simulink model "crane_DevDriv_2016a"  (R2016a)
settings: Solver=ode5  StartTime=0.0  StopTime=inf  FixedStep=0.01  RelTol=1e-3
values from neighbouring files (symbols this model uses):
  start_course = 1    [a_1_run_script.m]
  total_waypoints = length(waypoints_list)    [a_1_run_script.m]
undefined symbols (not defined in the file or in its folder): Crane3D_RangeBit, Crane3D_ScaleCoeff, xwaypoints, ywaypoints
undefined symbols (not defined in the file): RTDAC4PCIBaseAddress
libraries: simulink x2
settings Model: SimulationMode=external  ExtModeTrigDuration=5000  Creator=The MathWorks Inc.  LastModifiedBy=nadeen
settings DataIOCC: SaveFormat=StructureWithTime  SignalLoggingSaveFormat=ModelDataLogs  SignalLoggingName=logsOut
settings OptimizationCC: ExpressionDepthLimit=2147483647  InitFltsAndDblsToZero=on  EfficientMapNaN2IntZero=off
settings DebuggingCC: UnderspecifiedInitializationDetection=Classic  MergeDetectMultiDrivingBlocksExec=none  SignalResolutionControl=TryResolveAllWithWarning  FcnCallInpInsideContextMsg=EnableAllAsWarning  StateNameClashWarn=warning
settings HardwareCC: TargetBitPerLong=64  TargetBitPerPointer=64  TargetIntDivRoundTo=Zero  TargetEndianess=LittleEndian  TargetWordSize=64  TargetHWDeviceType=Intel->x86-64
settings ModelReferenceCC: PropagateSignalLabelsOutOfModel=off
settings RTWCC: SystemTargetFile=sldrt.tlc  TemplateMakefile=sldrt.tmf  Description=Simulink Desktop Real-Time  RTWCompilerOptimization=on
settings CodeAppCC: MaxIdLength=95
settings SimulinkDesktopRealTimeCC: TargetPreCompLibLocation=C:\Program Files\MATLAB\R2016b\toolbox\sldrt\lib\win64  TargetLangStandard=C89/C90 (ANSI)  SupportVariableSizeSignals=off
settings ConfigComp: CovSFcnEnable=off

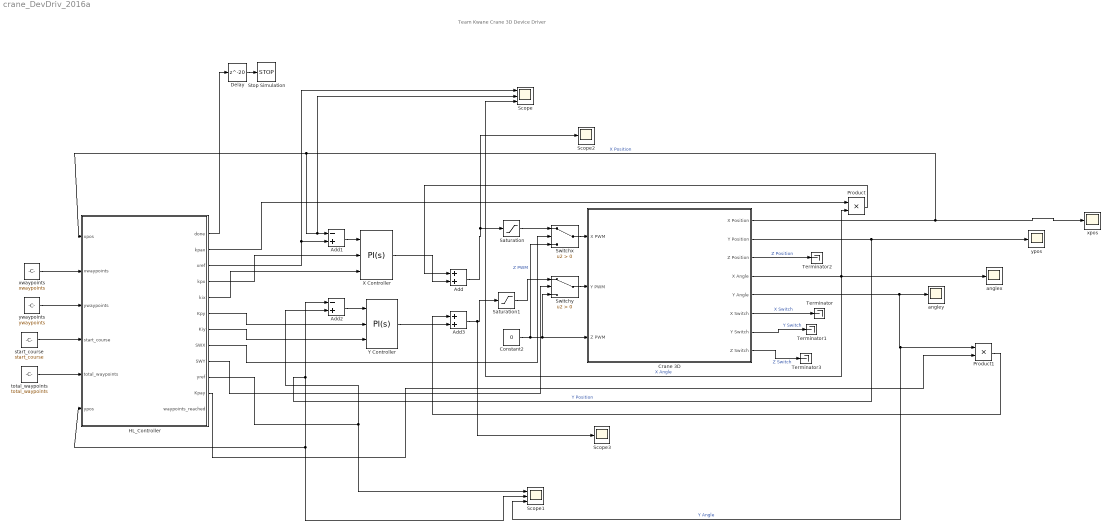
== system crane_DevDriv_2016a ==
  note: Team Kwane Crane 3D Device Driver
  Add : Sum
  Add1 : Sum  Inputs=-+
  Add2 : Sum  Inputs=-+
  Add3 : Sum
  Constant2 : Constant  Value=0
  Crane 3D : Subsystem  mask{BaseAddress=RTDAC4PCIBaseAddress, T0=0.01}
      mask prompts: BaseAddress "Base Address:"; T0 "Samping Period:"
      mask Display: image(imread('crane.jpeg'))
  Delay : Delay  DelayLength=20
  HL_Controller : Stateflow chart  TreatAsAtomicUnit=on
      settings: PermitHierarchicalResolution=ParametersOnly
  Product : Product
  Product1 : Product
  Saturation : Saturate  UpperLimit=0.8  LowerLimit=-0.8
  Saturation1 : Saturate  UpperLimit=0.8  LowerLimit=-0.8
  Scope : Scope  NumInputPorts=3
  Scope1 : Scope  NumInputPorts=3
  Scope2 : Scope
  Scope3 : Scope
  Stop Simulation : Stop
  Switchx : Switch  Criteria=u2 > Threshold
  Switchy : Switch  Criteria=u2 > Threshold
  Terminator{,1..3} (4 alike) : Terminator
  X Controller : simulink/Continuous/PID Controller  Controller=PI  TimeDomain=Continuous-time  SampleTime=-1  IntegratorMethod=Forward Euler  FilterMethod=Forward Euler  Form=Parallel  UseFilter=on  ControllerParametersSource=external  P=1  I=1  D=0  N=100  InitialConditionSource=internal  InitialConditionForIntegrator=0  InitialConditionForFilter=0  ExternalReset=none  LimitOutput=off  UpperSaturationLimit=inf  LowerSaturationLimit=-inf  LinearizeAsGain=on  AntiWindupMode=none  Kb=1  TrackingMode=off  Kt=1  PParamMin=[]  PParamMax=[]  IParamMin=[]  IParamMax=[]  DParamMin=[]  DParamMax=[]  NParamMin=[]  NParamMax=[]  KbParamMin=[]  KbParamMax=[]  KtParamMin=[]  KtParamMax=[]  POutMin=[]  POutMax=[]  IOutMin=[]  IOutMax=[]  DOutMin=[]  DOutMax=[]  NOutMin=[]  NOutMax=[]  KbOutMin=[]  KbOutMax=[]  KtOutMin=[]  KtOutMax=[]  IntegratorOutMin=[]  IntegratorOutMax=[]  FilterOutMin=[]  FilterOutMax=[]  SumOutMin=[]  SumOutMax=[]  SumI1OutMin=[]  SumI1OutMax=[]  SumI2OutMin=[]  SumI2OutMax=[]  SumI3OutMin=[]  SumI3OutMax=[]  SumDOutMin=[]  SumDOutMax=[]  SaturationOutMin=[]  SaturationOutMax=[]  IntegratorContinuousStateAttributes=''  IntegratorStateMustResolveToSignalObject=off  IntegratorRTWStateStorageClass=Auto  FilterContinuousStateAttributes=''  FilterStateMustResolveToSignalObject=off  FilterRTWStateStorageClass=Auto  DifferentiatorICPrevScaledInput=0  DifferentiatorOutMin=[]  DifferentiatorOutMax=[]
  Y Controller : simulink/Continuous/PID Controller  Controller=PI  TimeDomain=Continuous-time  SampleTime=-1  IntegratorMethod=Forward Euler  FilterMethod=Forward Euler  Form=Parallel  UseFilter=on  ControllerParametersSource=external  P=1  I=1  D=0  N=100  InitialConditionSource=internal  InitialConditionForIntegrator=0  InitialConditionForFilter=0  ExternalReset=none  LimitOutput=off  UpperSaturationLimit=inf  LowerSaturationLimit=-inf  LinearizeAsGain=on  AntiWindupMode=none  Kb=1  TrackingMode=off  Kt=1  PParamMin=[]  PParamMax=[]  IParamMin=[]  IParamMax=[]  DParamMin=[]  DParamMax=[]  NParamMin=[]  NParamMax=[]  KbParamMin=[]  KbParamMax=[]  KtParamMin=[]  KtParamMax=[]  POutMin=[]  POutMax=[]  IOutMin=[]  IOutMax=[]  DOutMin=[]  DOutMax=[]  NOutMin=[]  NOutMax=[]  KbOutMin=[]  KbOutMax=[]  KtOutMin=[]  KtOutMax=[]  IntegratorOutMin=[]  IntegratorOutMax=[]  FilterOutMin=[]  FilterOutMax=[]  SumOutMin=[]  SumOutMax=[]  SumI1OutMin=[]  SumI1OutMax=[]  SumI2OutMin=[]  SumI2OutMax=[]  SumI3OutMin=[]  SumI3OutMax=[]  SumDOutMin=[]  SumDOutMax=[]  SaturationOutMin=[]  SaturationOutMax=[]  IntegratorContinuousStateAttributes=''  IntegratorStateMustResolveToSignalObject=off  IntegratorRTWStateStorageClass=Auto  FilterContinuousStateAttributes=''  FilterStateMustResolveToSignalObject=off  FilterRTWStateStorageClass=Auto  DifferentiatorICPrevScaledInput=0  DifferentiatorOutMin=[]  DifferentiatorOutMax=[]
  anglex : Scope
  angley : Scope
  start_course : Constant  Value=start_course
  "total_waypoints " : Constant  Value=total_waypoints
  xpos : Scope
  xwaypoints : Constant  Value=xwaypoints
  ypos : Scope
  "ywaypoints " : Constant  Value=ywaypoints
  wires:
  Crane 3D/6(X Switch) -> Terminator/1  "X Switch"
  Crane 3D/7(Y Switch) -> Terminator1/1  "Y Switch"
  Crane 3D/8(Z Switch) -> Terminator3/1  "Z Switch"
  Crane 3D/1(X Position) -> Scope/2, Add1/1, HL_Controller/1(xpos), xpos/1  "X Position"
  Crane 3D/2(Y Position) -> Add2/1, HL_Controller/6(ypos), Scope1/2, ypos/1  "Y Position"
  Crane 3D/3(Z Position) -> Terminator2/1  "Z Position"
  Crane 3D/4(X Angle) -> Product/2, Scope/3, anglex/1  "X Angle"
  Crane 3D/5(Y Angle) -> Scope1/3, Product1/1, angley/1  "Y Angle"
  Constant2/1 -> Switchx/3, Switchy/3, Crane 3D/3(Z PWM)  "Z PWM"
  X Controller/1 -> Add/2
  Product/1 -> Add/1
  HL_Controller/2(kpax) -> Product/1
  Add/1 -> Scope2/1, Saturation/1
  HL_Controller/3(xref) -> Scope/1, Add1/2
  Add1/1 -> X Controller/1
  HL_Controller/10(yref) -> Scope1/1, Add2/2
  HL_Controller/11(Kpay) -> Product1/2
  Product1/1 -> Add3/1
  Add3/1 -> Scope3/1, Saturation1/1
  Y Controller/1 -> Add3/2
  HL_Controller/1(done) -> Delay/1
  Delay/1 -> Stop Simulation/1
  HL_Controller/4(kpx) -> X Controller/2
  HL_Controller/5(kix) -> X Controller/3
  Add2/1 -> Y Controller/1
  HL_Controller/6(Kpy) -> Y Controller/2
  HL_Controller/7(Kiy) -> Y Controller/3
  Saturation/1 -> Switchx/1
  Switchx/1 -> Crane 3D/1(X PWM)
  Saturation1/1 -> Switchy/1
  Switchy/1 -> Crane 3D/2(Y PWM)
  HL_Controller/8(SWX) -> Switchx/2
  HL_Controller/9(SWY) -> Switchy/2
  xwaypoints/1 -> HL_Controller/2(xwaypoints)
  "ywaypoints "/1 -> HL_Controller/3(ywaypoints)
  start_course/1 -> HL_Controller/4(start_course)
  "total_waypoints "/1 -> HL_Controller/5(total_waypoints)

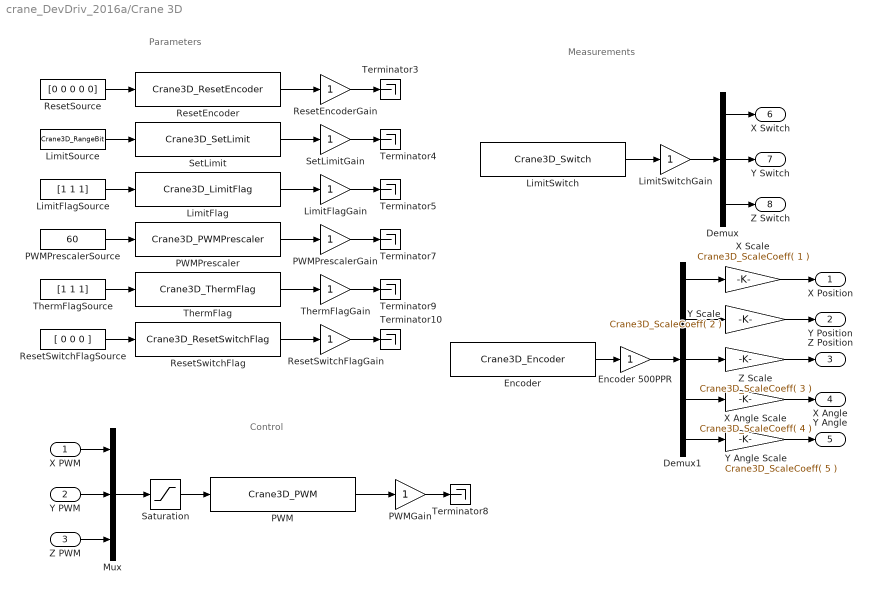
== system crane_DevDriv_2016a/Crane 3D ==
  note: Measurements
  note: Control
  note: Parameters
  X PWM : Inport
  Y PWM : Inport  Port=2
  Z PWM : Inport  Port=3
  Demux : Demux  Outputs=3
  Demux1 : Demux  Outputs=5
  Encoder : S-Function  FunctionName=Crane3D_Encoder  Parameters=BaseAddress, T0  SFunctionDeploymentMode=off  EnableBusSupport=off
  Encoder 500PPR : Gain  SaturateOnIntegerOverflow=on  OutDataTypeStr=Inherit: Same as input  ParamDataTypeStr=Inherit: Same as input
  LimitFlag : S-Function  FunctionName=Crane3D_LimitFlag  Parameters=BaseAddress, T0  SFunctionDeploymentMode=off  EnableBusSupport=off
  LimitFlagGain : Gain  SaturateOnIntegerOverflow=on  OutDataTypeStr=Inherit: Same as input  ParamDataTypeStr=Inherit: Same as input
  LimitFlagSource : Constant  Value=[1 1 1]
  LimitSource : Constant  Value=Crane3D_RangeBit
  LimitSwitch : S-Function  FunctionName=Crane3D_Switch  Parameters=BaseAddress, T0  SFunctionDeploymentMode=off  EnableBusSupport=off
  LimitSwitchGain : Gain  SaturateOnIntegerOverflow=on  OutDataTypeStr=Inherit: Same as input  ParamDataTypeStr=Inherit: Same as input
  Mux : Mux  Inputs=3
  PWM : S-Function  FunctionName=Crane3D_PWM  Parameters=BaseAddress, T0  SFunctionDeploymentMode=off  EnableBusSupport=off
  PWMGain : Gain  SaturateOnIntegerOverflow=on  OutDataTypeStr=Inherit: Same as input  ParamDataTypeStr=Inherit: Same as input
  PWMPrescaler : S-Function  FunctionName=Crane3D_PWMPrescaler  Parameters=BaseAddress, T0  SFunctionDeploymentMode=off  EnableBusSupport=off
  PWMPrescalerGain : Gain  SaturateOnIntegerOverflow=on  OutDataTypeStr=Inherit: Same as input  ParamDataTypeStr=Inherit: Same as input
  PWMPrescalerSource : Constant  Value=60
  ResetEncoder : S-Function  FunctionName=Crane3D_ResetEncoder  Parameters=BaseAddress, T0  SFunctionDeploymentMode=off  EnableBusSupport=off
  ResetEncoderGain : Gain  SaturateOnIntegerOverflow=on  OutDataTypeStr=Inherit: Same as input  ParamDataTypeStr=Inherit: Same as input
  ResetSource : Constant  Value=[0 0 0 0 0]
  "ResetSwitchFlag " : S-Function  FunctionName=Crane3D_ResetSwitchFlag  Parameters=BaseAddress, T0  SFunctionDeploymentMode=off  EnableBusSupport=off
  ResetSwitchFlagGain : Gain  SaturateOnIntegerOverflow=on  OutDataTypeStr=Inherit: Same as input  ParamDataTypeStr=Inherit: Same as input
  ResetSwitchFlagSource : Constant  Value=[ 0 0 0 ]
  Saturation : Saturate  UpperLimit=1  LowerLimit=-1
  SetLimit : S-Function  FunctionName=Crane3D_SetLimit  Parameters=BaseAddress, T0  SFunctionDeploymentMode=off  EnableBusSupport=off
  SetLimitGain : Gain  SaturateOnIntegerOverflow=on  OutDataTypeStr=Inherit: Same as input  ParamDataTypeStr=Inherit: Same as input
  Terminator{3..5,7..10} (7 alike) : Terminator
  "ThermFlag " : S-Function  FunctionName=Crane3D_ThermFlag  Parameters=BaseAddress, T0  SFunctionDeploymentMode=off  EnableBusSupport=off
  ThermFlagGain : Gain  SaturateOnIntegerOverflow=on  OutDataTypeStr=Inherit: Same as input  ParamDataTypeStr=Inherit: Same as input
  ThermFlagSource : Constant  Value=[1 1 1]
  X Angle Scale : Gain  Gain=Crane3D_ScaleCoeff( 4 )  OutDataTypeStr=Inherit: Same as input  ParamDataTypeStr=Inherit: Same as input
  X Scale : Gain  Gain=Crane3D_ScaleCoeff( 1 )  OutDataTypeStr=Inherit: Same as input  ParamDataTypeStr=Inherit: Same as input
  Y Angle Scale : Gain  Gain=Crane3D_ScaleCoeff( 5 )  OutDataTypeStr=Inherit: Same as input  ParamDataTypeStr=Inherit: Same as input
  Y Scale : Gain  Gain=Crane3D_ScaleCoeff( 2 )  OutDataTypeStr=Inherit: Same as input  ParamDataTypeStr=Inherit: Same as input
  Z Scale : Gain  Gain=Crane3D_ScaleCoeff( 3 )  OutDataTypeStr=Inherit: Same as input  ParamDataTypeStr=Inherit: Same as input
  X Position : Outport  InitialOutput=0
  Y Position : Outport  Port=2  InitialOutput=0
  Z Position : Outport  Port=3  InitialOutput=0
  X Angle : Outport  Port=4  InitialOutput=0
  Y Angle : Outport  Port=5  InitialOutput=0
  X Switch : Outport  Port=6  InitialOutput=0
  Y Switch : Outport  Port=7  InitialOutput=0
  Z Switch : Outport  Port=8  InitialOutput=0
  wires:
  Demux1/1 -> X Scale/1
  Demux1/2 -> Y Scale/1
  Demux1/3 -> Z Scale/1
  Demux1/4 -> X Angle Scale/1
  Demux1/5 -> Y Angle Scale/1
  X Angle Scale/1 -> X Angle/1
  Y Angle Scale/1 -> Y Angle/1
  Y Scale/1 -> Y Position/1
  X Scale/1 -> X Position/1
  Z Scale/1 -> Z Position/1
  Demux/3 -> Z Switch/1
  Demux/2 -> Y Switch/1
  Demux/1 -> X Switch/1
  LimitSwitchGain/1 -> Demux/1
  LimitSwitch/1 -> LimitSwitchGain/1
  X PWM/1 -> Mux/1
  Y PWM/1 -> Mux/2
  Z PWM/1 -> Mux/3
  ResetSwitchFlagGain/1 -> Terminator10/1
  ThermFlagGain/1 -> Terminator9/1
  PWMPrescalerGain/1 -> Terminator7/1
  LimitFlagGain/1 -> Terminator5/1
  SetLimitGain/1 -> Terminator4/1
  ResetEncoderGain/1 -> Terminator3/1
  ResetSwitchFlagSource/1 -> "ResetSwitchFlag "/1
  ThermFlagSource/1 -> "ThermFlag "/1
  PWMPrescalerSource/1 -> PWMPrescaler/1
  LimitFlagSource/1 -> LimitFlag/1
  LimitSource/1 -> SetLimit/1
  ResetSource/1 -> ResetEncoder/1
  "ResetSwitchFlag "/1 -> ResetSwitchFlagGain/1
  "ThermFlag "/1 -> ThermFlagGain/1
  PWMPrescaler/1 -> PWMPrescalerGain/1
  LimitFlag/1 -> LimitFlagGain/1
  SetLimit/1 -> SetLimitGain/1
  ResetEncoder/1 -> ResetEncoderGain/1
  PWMGain/1 -> Terminator8/1
  PWM/1 -> PWMGain/1
  Mux/1 -> Saturation/1
  Saturation/1 -> PWM/1
  Encoder/1 -> Encoder 500PPR/1
  Encoder 500PPR/1 -> Demux1/1

== stateflow chart crane_DevDriv_2016a/HL_Controller ==
  note: Functions Used in FSM
  state S0_IDLE
    entry:
    xlocal=0;
    ylocal=0;
    done=false;
    index=1;
    Kp_l=0;
    Ki_l=0;
    Kpa_l=0;
    Kix_l=0;
    Kpx_l=0;
    Kpax_l=0;
    swx_l=0;
    swy_l=0;
    waypoints_reached_l=0;
  note: Dynamically set PI Parameters based on distance
  state func1_setpidx(xcurrent,xdest) [function]
    (default) -> (junction 3) : {[Kix_l,Kpax_l,Kpx_l,swx_l]=setpidx(xcurrent,xdest);}
  state S1_Initialize
    state S1_setpoints1 [parallel]
      entry:
      xlocal=xwaypoints(index);
      ylocal=ywaypoints(index);
      arrived=0;
      settings: executionOrder=1
    state S1_setup_pidy1 [parallel]
      entry:
      func1_setpidy(ypos,ywaypoints(index))
      settings: executionOrder=2
    state S1_setup_pidy [parallel]
      entry:
      func1_setpidx(xpos,xwaypoints(index))
      settings: executionOrder=3
  state func1_setpidy(ycurrent,ydest) [function]
    (default) -> (junction 32) : {[Kp_l,Ki_l,Kpa_l,swy_l]=setpidy(ycurrent,ydest);}
  state S2_Move_to_waypoint
    entry:
    xref=xlocal;
    yref=ylocal;
    Kpy=Kp_l;
    Kiy=Ki_l;
    Kpay=Kpa_l;
    kix=Kix_l;
    kpx=Kpx_l;
    kpax=Kpax_l;
    arrived=0;
    sustained=0;
    SWX=swx_l;
    SWY=swy_l;
  note: Waypoints Reached Stats
  state func2_CheckArrival(currentx,currenty,xdest,ydest) [function]
    (default) -> (junction 54) : % checks for steady state
    (junction 54) -> (junction 42) [order 1] : [abs(xdest-currentx)<0.004&& abs(ydest-currenty)<0.004]
    (junction 54) -> (junction 44) [order 2] : {arrived=0;}
    (junction 42) -> (junction 40) : {arrived=1;}
    (junction 40) -> (junction 44)
    (junction 44) -> (junction 55)
  state S3_wait_for_arrival
    entry:index=index+1;
    during: func2_CheckArrival(xpos,ypos,xlocal,ylocal)
  note: Check if all waypoints reached
  state func3_CheckDone(count,total) [function]
    (default) -> (junction 60)
    (junction 60) -> (junction 68) [order 1] : [count>total]
    (junction 60) -> (junction 69) [order 2] : {finished=0;}
    (junction 68) -> (junction 70) : {finished=1;}
    (junction 70) -> (junction 69)
    (junction 69) -> (junction 71)
  state S4_checkifdone
    entry: func3_CheckDone(index,total_waypoints)
    waypoints_reached_l=waypoints_reached_l+arrived;
  state s3_delay
  state func4_CheckAngle(thetax,thetay) [function]
    (default) -> (junction 141) : % checks for steady state
    (junction 141) -> (junction 144) [order 1] : [abs(thetax)<=0.004&&abs(thetay)<=0.004]
    (junction 141) -> (junction 146) [order 2] : {sustained=0;}
    (junction 144) -> (junction 142) : {sustained=1;}
    (junction 142) -> (junction 146)
    (junction 146) -> (junction 137)
  state S5_done
    entry:
    SWX=0;
    SWY=0;
    done=true;
    waypoints_reached=waypoints_reached_l;
  (default) -> S0_IDLE
  S0_IDLE -> S1_Initialize : [start_course==1]
  S4_checkifdone -> S1_Initialize [order 2] : [finished==0]
  S1_Initialize -> S2_Move_to_waypoint
  S2_Move_to_waypoint -> S3_wait_for_arrival
  S3_wait_for_arrival -> s3_delay [order 2] : [arrived==1]
  S3_wait_for_arrival -> S4_checkifdone [order 1] : [after(7,sec)]
  s3_delay -> S4_checkifdone
  S4_checkifdone -> S5_done [order 1] : [finished==1]
  data: Kix function_output; Kpax function_output; xcurrent function_input; xdest function_input; Kpx function_output; swx function_output; xcurrent function_input; xdest function_input; Kp function_output; ycurrent function_input; ydest function_input; Ki function_output; Kpa function_output; swy function_output; ycurrent function_input; ydest function_input; currentx function_input; currenty function_input; xdest function_input; ydest function_input; count function_input; total function_input; thetax function_input; thetay function_input; xpos input; xwaypoints input; ywaypoints input; start_course input; total_waypoints input; ypos input; finished local; done output; kpax output; xref output; kpx output; kix output; Kpy output; Kiy output; SWX output; SWY output; yref output; Kpay output; waypoints_reached output; xlocal local; ylocal local; Ki_l local; Kpx_l local; Kpa_l local; index local; Kp_l local; Kpax_l local; Kix_l local; arrived local; waypoints_reached_l local; swx_l local; swy_l local; sustained local
  function [Kix,Kpax,Kpx,swx]= setpidx(xcurrent,xdest):
    | function [Kix,Kpax,Kpx,swx]= setpidx(xcurrent,xdest)
    | 	swx=1;
    |   temp=abs(xcurrent-xdest);
    | 	if temp<=0.005
    | 		swx=0;
    | 		Kix=0.;
    | 		Kpx=0;
    | 		Kpax=0;
    | elseif temp<=0.02
    | 			Kix=0.0;
    | 		Kpx=30;
    | 		Kpax=5.5;
    | elseif temp<=0.04
    | 		Kix=0.01;
    | 		Kpx=17;
    | 		Kpax=7;
    | elseif temp<=0.06
    | 			Kix=0.2;
    | 		Kpx=9.5;
    | 		Kpax=6;
    | elseif temp<=0.08
    | 		Kix=0.01;
    | 		Kpx=7.5;
    | 		Kpax=6;
    | elseif temp<=0.09
    | Kix=0.1;
    | Kpx=6.8;
    | Kpax=4;
    | elseif temp<=0.10
    | Kix=0.08;
    | Kpx=6.2;
    | Kpax=4.6;
    | elseif temp<=0.11
    | Kix=0.25;
    | Kpx=5.8;
    | Kpax=3.4;
    | %tsx=3.5
    | elseif temp<=0.12
    | Kix=0.15;
    | Kpx=5.6;
    | Kpax=3.4;
    | %tsx=3
    | elseif temp<=0.15
    | Kix=0.05;
    | Kpx=5.2;
    | Kpax=4.1;
    | elseif temp<=0.18
    | Kix=0.02;
    | Kpx=4.6;
    | Kpax=4.4;	
    | elseif temp<=0.20
    | Kix=0.005;
    | Kpx=4.42;
    | Kpax=4.4;
    | elseif temp<=0.23
    | Kix=0.02;
    | Kpx=4;
    | Kpax=5.2;	
    | elseif temp<=0.25
    | Kix=0.02;
    | Kpx=3.8;
    | Kpax=5.2;
    | elseif temp<=0.28
    | 		Kix=0.01;
    | 		Kpx=3.7;
    | 		Kpax=5.2;	
    | elseif temp<=0.30
    | 		Kix=0.01;
    | 		Kpx=3.6;
    | 		Kpax=5;
    | 	elseif temp<=0.33
    | 		Kix=0.00;
    | 		Kpx=3.5;
    | 		Kpax=5.6;
    | 		elseif temp<=0.35
    | 		Kix=0.005;
    | 		Kpx=3.4;
    | 		Kpax=5.2;
    | 		elseif temp<=0.40
    | 		Kix=0.01;
    | 		Kpx=3.2;
    | 		Kpax=5.8;
    | 		elseif temp<=0.42
    | 		Kix=0.01;
    | 		Kpx=3.2;
    | 		Kpax=5.4;
    | 		elseif temp<=0.47
    | 		Kix=0.005;
    | 		Kpx=3.2;
    | 		Kpax=5.4;
    | 	else
    | 		swx=0;
    | 		Kix=0.;
    | 		Kpx=0;
    | 		Kpax=0;
    | 		
    | 	end
  function [Kp,Ki,Kpa,swy]= setpidy(ycurrent,ydest):
    | function [Kp,Ki,Kpa,swy]= setpidy(ycurrent,ydest)
    | 	swy=1;
    |   temp=abs(ycurrent-ydest);
    | 	if temp<=0.005
    | 		Kp=0;
    | 		Ki=0;
    | 		Kpa=0;
    | 		swy=0;
    | elseif temp<=0.02
    | 	Ki=2.8;
    | 		Kp=29;
    | 		Kpa=7.5;
    | elseif temp<=0.04
    | 	Ki=0.01;
    | 		Kp=13.;
    | 		Kpa=7.5;
    | elseif temp<=0.06
    | 			Ki=0.2;
    | 		Kp=8.2;
    | 		Kpa=5.2;
    | elseif temp<=0.08
    | 	Ki=0.05;
    | 		Kp=6.6;
    | 		Kpa=4.2;
    | elseif temp<=0.09
    | Ki=0.1;
    | Kp=5.8;
    | Kpa=3;
    | elseif temp<=0.10
    | Ki=0.02;
    | Kp=5.4;
    | Kpa=4.05;
    | elseif temp<=0.11
    | Ki=0.01;
    | Kp=5.1;
    | Kpa=3.4;
    | %tsy=3.5
    | elseif temp<=0.12
    | Ki=0.01;
    | Kp=5.1;
    | Kpa=3.4;
    | %tsy=3.5
    | elseif temp<=0.15
    | Ki=0.02;
    | Kp=4.5;
    | Kpa=4.2;
    | elseif temp<=0.18
    | Ki=0.02;
    | Kp=4.2;
    | Kpa=3.6;	
    | elseif temp<=0.20
    | Ki=0.025;
    | Kp=3.9;
    | Kpa=3.6;
    | elseif temp<=0.23
    | Ki=0.01;
    | Kp=3.6;
    | Kpa=5;		
    | 	elseif temp<=0.25
    | Ki=0.01;
    | Kp=3.4;
    | Kpa=5;
    | elseif temp<=0.28
    | 		Ki=0.01;
    | 		Kp=3.4;
    | 		Kpa=5.2;
    | elseif temp<=0.30
    | 		Ki=0.01;
    | 		Kp=3.2;
    | 		Kpa=5;
    | elseif temp<=0.33
    | 		Ki=0.002;
    | 		Kp=3.2;
    | 		Kpa=5.2;	
    | elseif temp<=0.35
    | 		Ki=0.01;
    | 		Kp=3.0;
    | 		Kpa=5.5;
    | elseif temp<=0.40	
    | 		Ki=0.01;
    | 		Kp=3.;
    | 		Kpa=5.6;
    | elseif temp<=0.42
    | 		Ki=0.01;
    | 		Kp=3.0;
    | 		Kpa=5.2;
    | 	elseif temp<=0.47
    | 		Ki=0.012;
    | 		Kp=2.9;
    | 		Kpa=5.2;
    | 	else
    | 		Kp=0;
    | 		Ki=0;
    | 		Kpa=0;
    | 		swy=0;	
    | 	end
